simulink model "TST_IAirHt_VD"  (R2016b)
settings: Solver=FixedStepDiscrete  StartTime=0.0  StopTime=simTime  FixedStep=sampleTime  RelTol=1e-3
values from neighbouring files (symbols this model uses):
  testCase = 1    [initTST_IAirHt_VD_001.m]
libraries: simulink x3, UnitTest_Lib x1
settings Model: Creator=zhengjinyan  LastModifiedBy=zhengjinyan
settings DebuggingCC: SignalRangeChecking=error

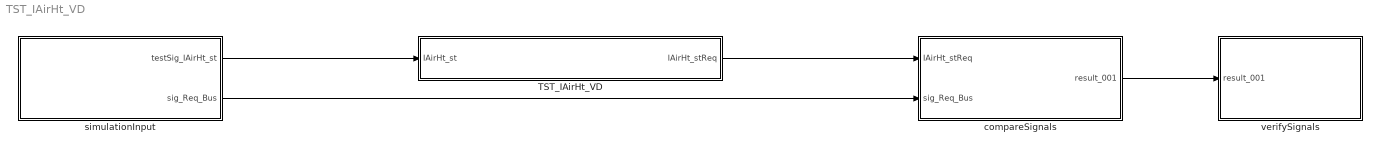
== system TST_IAirHt_VD ==
  TST_IAirHt_VD : Subsystem
  compareSignals : Subsystem
  simulationInput : Subsystem
  verifySignals : Subsystem
  wires:
  simulationInput/1(testSig_IAirHt_st) -> TST_IAirHt_VD/1(IAirHt_st)
  TST_IAirHt_VD/1(IAirHt_stReq) -> compareSignals/1(IAirHt_stReq)
  simulationInput/2(sig_Req_Bus) -> compareSignals/2(sig_Req_Bus)
  compareSignals/1(result_001) -> verifySignals/1(result_001)

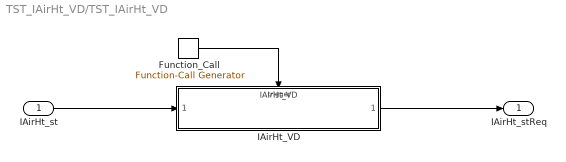
== system TST_IAirHt_VD/TST_IAirHt_VD ==
  IAirHt_st : Inport
  Function_Call : simulink/Ports & Subsystems/Function-Call Generator  sample_time=sampleTime  numberOfIterations=1
  IAirHt_VD : ModelReference  ModelNameDialog=IAirHt_VD  SimulationMode=Normal  ModelReferenceVersion=1.2  TriggerPortName=function  TriggerPortTriggerType=function-call  TriggerPortStatesWhenEnabling=held
  IAirHt_stReq : Outport
  wires:
  Function_Call/1 -> IAirHt_VD/Trigger
  IAirHt_st/1 -> IAirHt_VD/1
  IAirHt_VD/1 -> IAirHt_stReq/1

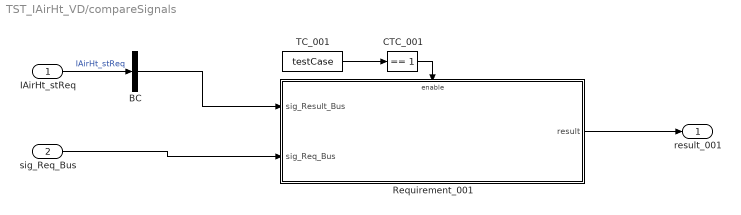
== system TST_IAirHt_VD/compareSignals ==
  IAirHt_stReq : Inport
  sig_Req_Bus : Inport  Port=2
  BC : BusCreator  Inputs=1
  CTC_001 : simulink/Logic and Bit Operations/Compare To Constant  relop===  const=1  OutDataTypeStr=boolean
  Requirement_001 : Subsystem
  TC_001 : Constant  Value=testCase
  result_001 : Outport
  wires:
  IAirHt_stReq/1 -> BC/1  "IAirHt_stReq"
  TC_001/1 -> CTC_001/1
  CTC_001/1 -> Requirement_001/Enable
  sig_Req_Bus/1 -> Requirement_001/2(sig_Req_Bus)
  BC/1 -> Requirement_001/1(sig_Result_Bus)
  Requirement_001/1(result) -> result_001/1

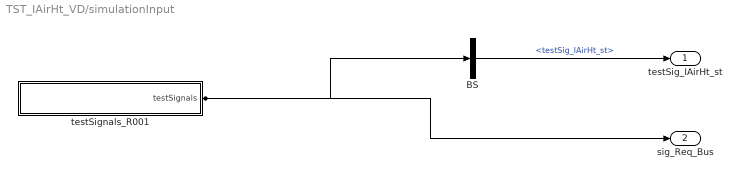
== system TST_IAirHt_VD/simulationInput ==
  BS : BusSelector  OutputSignals=testSig_IAirHt_st
  testSignals_R001 : Subsystem
  testSig_IAirHt_st : Outport
  sig_Req_Bus : Outport  Port=2
  wires:
  BS/1 -> testSig_IAirHt_st/1  "<testSig_IAirHt_st>"
  testSignals_R001/1(testSignals) -> BS/1, sig_Req_Bus/1

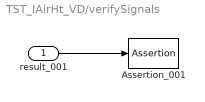
== system TST_IAirHt_VD/verifySignals ==
  result_001 : Inport
  Assertion_001 : Assertion  Enabled=off
  wires:
  result_001/1 -> Assertion_001/1

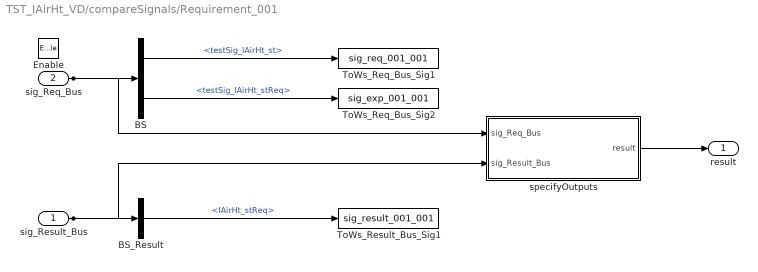
== system TST_IAirHt_VD/compareSignals/Requirement_001 ==
  sig_Result_Bus : Inport
  sig_Req_Bus : Inport  Port=2
  Enable : EnablePort
  BS : BusSelector  OutputSignals=testSig_IAirHt_st,testSig_IAirHt_stReq
  BS_Result : BusSelector  OutputSignals=IAirHt_stReq
  ToWs_Req_Bus_Sig1 : ToWorkspace  VariableName=sig_req_001_001  SaveFormat=Structure With Time
  ToWs_Req_Bus_Sig2 : ToWorkspace  VariableName=sig_exp_001_001  SaveFormat=Structure With Time
  ToWs_Result_Bus_Sig1 : ToWorkspace  VariableName=sig_result_001_001  SaveFormat=Structure With Time
  specifyOutputs : Subsystem
  result : Outport
  wires:
  sig_Req_Bus/1 -> BS/1, specifyOutputs/1(sig_Req_Bus)
  BS/1 -> ToWs_Req_Bus_Sig1/1  "<testSig_IAirHt_st>"
  BS/2 -> ToWs_Req_Bus_Sig2/1  "<testSig_IAirHt_stReq>"
  sig_Result_Bus/1 -> BS_Result/1, specifyOutputs/2(sig_Result_Bus)
  BS_Result/1 -> ToWs_Result_Bus_Sig1/1  "<IAirHt_stReq>"
  specifyOutputs/1(result) -> result/1

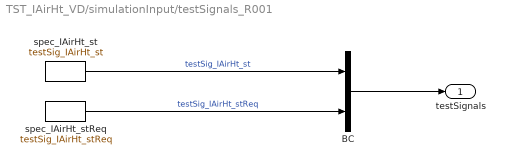
== system TST_IAirHt_VD/simulationInput/testSignals_R001 ==
  BC : BusCreator  Inputs=2
  spec_IAirHt_st : FromWorkspace  VariableName=testSig_IAirHt_st  Interpolate=off  OutputAfterFinalValue=Holding final value
  spec_IAirHt_stReq : FromWorkspace  VariableName=testSig_IAirHt_stReq  Interpolate=off  OutputAfterFinalValue=Holding final value
  testSignals : Outport
  wires:
  BC/1 -> testSignals/1
  spec_IAirHt_st/1 -> BC/1  "testSig_IAirHt_st"
  spec_IAirHt_stReq/1 -> BC/2  "testSig_IAirHt_stReq"

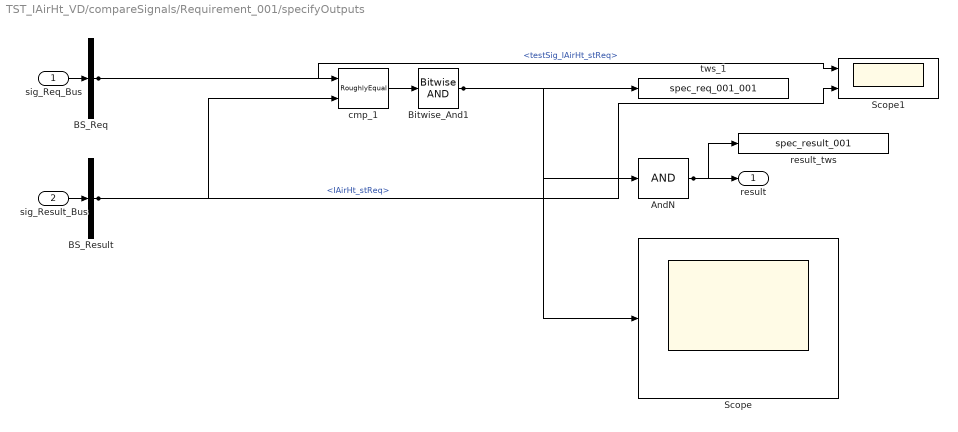
== system TST_IAirHt_VD/compareSignals/Requirement_001/specifyOutputs ==
  sig_Req_Bus : Inport
  sig_Result_Bus : Inport  Port=2
  AndN : Logic  Inputs=1
  BS_Req : BusSelector  OutputSignals=testSig_IAirHt_stReq
  BS_Result : BusSelector  OutputSignals=IAirHt_stReq
  Bitwise_And1 : simulink/Logic and Bit Operations/Bitwise Operator  logicop=AND  UseBitMask=off  BitMask=bin2dec('11011001')  BitMaskRealWorld=Stored Integer
  Scope : Scope
  Scope1 : Scope  NumInputPorts=2
  cmp_1 : UnitTest_Lib/RoughlyEqual  slope=0.1
  result_tws : ToWorkspace  VariableName=spec_result_001
  tws_1 : ToWorkspace  VariableName=spec_req_001_001
  result : Outport
  wires:
  sig_Req_Bus/1 -> BS_Req/1
  sig_Result_Bus/1 -> BS_Result/1
  AndN/1 -> result/1, result_tws/1
  BS_Req/1 -> cmp_1/1, Scope1/1  "<testSig_IAirHt_stReq>"
  BS_Result/1 -> cmp_1/2, Scope1/2  "<IAirHt_stReq>"
  cmp_1/1 -> Bitwise_And1/1
  Bitwise_And1/1 -> tws_1/1, AndN/1, Scope/1
